simulink model "PTEngineCU"  (Simulink 7.5)
settings: Solver=ode45  StartTime=0.0  StopTime=inf  RelTol=1e-3
PreLoadFcn:
  | Trq_x = [500.0, 600.0, 700.0, 800.0, 1000.0, 2000.0, 3000.0, 4000.0, 4500.0, 5000.0, 6000.0, 7000.0, 8000.0];
  | TrqFull_y = [10.0, 40.0, 70.0, 95.0, 120.0, 145.0, 165.0, 180.0, 185.0, 182.0, 168.0, 130.0, 0.0];
  | 
  | TrqDrag_y = [-10.0, -10.0, -10.0, -10.0, -10.0, -20.0, -30.0, -40.0, -45.0, -50.0, -60.0, -70.0, -80.0];
  | 
  | TrqOpt_y = [0.0, 0.0, 0.0, 0.0, 0.0, 0.0, 0.0, 0.0, 0.0, 0.0, 0.0, 0.0, 0.0];
InitFcn:
  | Trq_x = [500.0, 600.0, 700.0, 800.0, 1000.0, 2000.0, 3000.0, 4000.0, 4500.0, 5000.0, 6000.0, 7000.0, 8000.0];
  | TrqFull_y = [10.0, 40.0, 70.0, 95.0, 120.0, 145.0, 165.0, 180.0, 185.0, 182.0, 168.0, 130.0, 0.0];
  | 
  | TrqDrag_y = [-10.0, -10.0, -10.0, -10.0, -10.0, -20.0, -30.0, -40.0, -45.0, -50.0, -60.0, -70.0, -80.0];
  | 
  | TrqOpt_y = [0.0, 0.0, 0.0, 0.0, 0.0, 0.0, 0.0, 0.0, 0.0, 0.0, 0.0, 0.0, 0.0];
libraries: simulink x8, CarMaker4SL x5
(part 2 of 2)

== system PTEngineCU/CarMaker/IPG Vehicle/CarAndTrailer/Forces/Vehicle Forces ==
  Sync_In : Inport  OutDataType=sfix(16)  OutScaling=2^0
  Bus Creator1 : BusCreator  Inputs=12
  Bus Creator5 : BusCreator  Inputs=13
  Bus Creator8 : BusCreator  Inputs=16
  Demux : Demux  Outputs=16
  Demux1 : Demux  Outputs=12
  Demux5 : Demux  Outputs=13
  Forces : S-Function  FunctionName=CM_Sfun  Parameters='Forces'  EnableBusSupport=off
  Sync_Out : Outport  OutDataType=sfix(16)  OutScaling=2^0
  Car.Virtual : Outport  Port=2  OutDataType=sfix(16)  OutScaling=2^0
  Car.Aero : Outport  Port=3  OutDataType=sfix(16)  OutScaling=2^0
  Car.Load : Outport  Port=4  OutDataType=sfix(16)  OutScaling=2^0
  wires:
  Demux5/7 -> Bus Creator5/7  "car Aero vRes_1 z"
  Demux5/6 -> Bus Creator5/6  "car Aero vRes_1 y"
  Demux5/5 -> Bus Creator5/5  "car Aero vRes_1 x"
  Demux5/4 -> Bus Creator5/4  "Vehicle Wind_vel_0 z"
  Demux5/3 -> Bus Creator5/3  "Vehicle Wind_vel_0 y"
  Demux5/2 -> Bus Creator5/2  "Vehicle Wind_vel_0 x"
  Demux5/1 -> Bus Creator5/1  "Vehicle sRoadAero"
  Demux5/8 -> Bus Creator5/8  "car Aero Frc_1 x"
  Demux5/9 -> Bus Creator5/9  "car Aero Frc_1 y"
  Demux5/10 -> Bus Creator5/10  "car Aero Frc_1 z"
  Demux5/13 -> Bus Creator5/13  "car Aero Trq_1 z"
  Demux5/12 -> Bus Creator5/12  "car Aero Trq_1 y"
  Demux5/11 -> Bus Creator5/11  "car Aero Trq_1 x"
  Forces/4 -> Demux/1
  Demux/12 -> Bus Creator8/12  "Car Load_2 tz"
  Demux/11 -> Bus Creator8/11  "Car Load_2 ty"
  Demux/10 -> Bus Creator8/10  "Car Load_2 tx"
  Demux/9 -> Bus Creator8/9  "Car Load_2 mass"
  Demux/8 -> Bus Creator8/8  "Car Load_1 tz"
  Demux/7 -> Bus Creator8/7  "Car Load_1 ty"
  Demux/6 -> Bus Creator8/6  "Car Load_1 tx"
  Demux/5 -> Bus Creator8/5  "Car Load_1 mass"
  Demux/4 -> Bus Creator8/4  "Car Load_0 tz"
  Demux/3 -> Bus Creator8/3  "Car Load_0 ty"
  Demux/2 -> Bus Creator8/2  "Car Load_0 tx"
  Demux/1 -> Bus Creator8/1  "Car Load_0 mass"
  Bus Creator8/1 -> Car.Load/1
  Bus Creator1/1 -> Car.Virtual/1
  Forces/2 -> Demux1/1
  Forces/3 -> Demux5/1
  Demux1/3 -> Bus Creator1/3  "Car Virtual Frc_1 z"
  Demux1/2 -> Bus Creator1/2  "Car Virtual Frc_1 y"
  Demux1/1 -> Bus Creator1/1  "Car Virtual Frc_1 x"
  Bus Creator5/1 -> Car.Aero/1
  Forces/1 -> Sync_Out/1
  Sync_In/1 -> Forces/1
  Demux1/4 -> Bus Creator1/4  "Car Virtual Frc_0 x"
  Demux1/5 -> Bus Creator1/5  "Car Virtual Frc_0 y"
  Demux1/6 -> Bus Creator1/6  "Car Virtual Frc_0 z"
  Demux1/7 -> Bus Creator1/7  "Car Virtual Trq_1 x"
  Demux1/8 -> Bus Creator1/8  "Car Virtual Trq_1 y"
  Demux1/9 -> Bus Creator1/9  "Car Virtual Trq_1 z"
  Demux1/10 -> Bus Creator1/10  "Car Virtual Trq_0 x"
  Demux1/11 -> Bus Creator1/11  "Car Virtual Trq_0 y"
  Demux1/12 -> Bus Creator1/12  "Car Virtual Trq_0 z"
  Demux/13 -> Bus Creator8/13  "Car Load_3 mass"
  Demux/14 -> Bus Creator8/14  "Car Load_3 tx"
  Demux/15 -> Bus Creator8/15  "Car Load_3 ty"
  Demux/16 -> Bus Creator8/16  "Car Load_3 tz"

== system PTEngineCU/CarMaker/IPG Vehicle/CarAndTrailer/Trailer/CreateBus Car.Hitch.FrcTrq ==
  In1 : Inport  OutDataType=sfix(16)  OutScaling=2^0
  Bus Creator7 : BusCreator  Inputs=6
  Demux7 : Demux  Outputs=6
  Car.Hitch.FrcTrq : Outport  OutDataType=sfix(16)  OutScaling=2^0
  wires:
  Demux7/1 -> Bus Creator7/1  "Car Hitch Frc2Car x"
  Demux7/2 -> Bus Creator7/2  "Car Hitch Frc2Car y"
  Demux7/3 -> Bus Creator7/3  "Car Hitch Frc2Car z"
  Demux7/4 -> Bus Creator7/4  "Car Hitch Trq2Car x"
  Demux7/5 -> Bus Creator7/5  "Car Hitch Trq2Car y"
  Demux7/6 -> Bus Creator7/6  "Car Hitch Trq2Car z"
  Bus Creator7/1 -> Car.Hitch.FrcTrq/1
  In1/1 -> Demux7/1

== system PTEngineCU/CarMaker/IPG Vehicle/CarAndTrailer/Trailer/CreateBus Vhcl.Motion ==
  In1 : Inport  OutDataType=sfix(16)  OutScaling=2^0
  Demux1 : Demux  Outputs=16
  Mux1 : Mux  Inputs=16
  Out1 : Outport  OutDataType=sfix(16)  OutScaling=2^0
  wires:
  Mux1/1 -> Out1/1
  In1/1 -> Demux1/1
  Demux1/16 -> Mux1/16  "Vhcl YawAcc"
  Demux1/15 -> Mux1/15  "Vhcl YawRate"
  Demux1/14 -> Mux1/14  "Vhcl Yaw"
  Demux1/13 -> Mux1/13  "Vhcl PitchAcc"
  Demux1/12 -> Mux1/12  "Vhcl PitchVel"
  Demux1/11 -> Mux1/11  "Vhcl Pitch"
  Demux1/10 -> Mux1/10  "Vhcl RollAcc"
  Demux1/9 -> Mux1/9  "Vhcl RollVel"
  Demux1/8 -> Mux1/8  "Vhcl Roll"
  Demux1/7 -> Mux1/7  "Vhcl Hitch_Pos z"
  Demux1/6 -> Mux1/6  "Vhcl Hitch_Pos y"
  Demux1/5 -> Mux1/5  "Vhcl Hitch_Pos x"
  Demux1/4 -> Mux1/4  "Vhcl sRoadAero"
  Demux1/3 -> Mux1/3  "Vhcl sRoad"
  Demux1/2 -> Mux1/2  "Vhcl Distance"
  Demux1/1 -> Mux1/1  "Vhcl v"

== system PTEngineCU/CarMaker/IPG Vehicle/CarAndTrailer/Trailer/CreateBus Vhcl.PoI ==
  In1 : Inport  OutDataType=sfix(16)  OutScaling=2^0
  Bus Creator3 : BusCreator  Inputs=18
  Demux3 : Demux  Outputs=18
  Out1 : Outport  OutDataType=sfix(16)  OutScaling=2^0
  wires:
  Demux3/1 -> Bus Creator3/1  "Vhcl PoI_Pos x"
  Bus Creator3/1 -> Out1/1
  In1/1 -> Demux3/1
  Demux3/2 -> Bus Creator3/2  "Vhcl PoI_Pos y"
  Demux3/3 -> Bus Creator3/3  "Vhcl PoI_Pos z"
  Demux3/4 -> Bus Creator3/4  "Vhcl PoI_Vel x"
  Demux3/5 -> Bus Creator3/5  "Vhcl PoI_Vel y"
  Demux3/6 -> Bus Creator3/6  "Vhcl PoI_Vel z"
  Demux3/7 -> Bus Creator3/7  "Vhcl PoI_Acc x"
  Demux3/8 -> Bus Creator3/8  "Vhcl PoI_Acc y"
  Demux3/9 -> Bus Creator3/9  "Vhcl PoI_Acc z"
  Demux3/10 -> Bus Creator3/10  "Vhcl PoI_Vel_1 x"
  Demux3/11 -> Bus Creator3/11  "Vhcl PoI_Vel_1 y"
  Demux3/12 -> Bus Creator3/12  "Vhcl PoI_Vel_1 z"
  Demux3/13 -> Bus Creator3/13  "Vhcl PoI_Acc_1 x"
  Demux3/14 -> Bus Creator3/14  "Vhcl PoI_Acc_1 y"
  Demux3/15 -> Bus Creator3/15  "Vhcl PoI_Acc_1 z"
  Demux3/16 -> Bus Creator3/16  "Vhcl PoI_GCS Long"
  Demux3/17 -> Bus Creator3/17  "Vhcl PoI_GCS Lat"
  Demux3/18 -> Bus Creator3/18  "Vhcl PoI_GCS Elev"

== system PTEngineCU/CarMaker/IPG Vehicle/CarAndTrailer/Trailer/CreateBus Vhcl.Steering ==
  In1 : Inport  OutDataType=sfix(16)  OutScaling=2^0
  Bus Creator3 : BusCreator
  Demux : Demux
  Out1 : Outport  OutDataType=sfix(16)  OutScaling=2^0
  wires:
  In1/1 -> Demux/1
  Demux/4 -> Bus Creator3/4  "Vhcl Steering Trq"
  Demux/2 -> Bus Creator3/2  "Vhcl Steering AngVel"
  Demux/3 -> Bus Creator3/3  "Vhcl Steering AngAcc"
  Demux/1 -> Bus Creator3/1  "Vhcl Steering Ang"
  Bus Creator3/1 -> Out1/1

== system PTEngineCU/CarMaker/IPG Vehicle/CarAndTrailer/Trailer/CreateBus Vhcl.Wheel.FL ==
  In1 : Inport  OutDataType=sfix(16)  OutScaling=2^0
  Bus Creator3 : BusCreator  Inputs=14
  Demux3 : Demux  Outputs=14
  Out1 : Outport  OutDataType=sfix(16)  OutScaling=2^0
  wires:
  Demux3/1 -> Bus Creator3/1  "Vhcl Wheel FL t x"
  Bus Creator3/1 -> Out1/1
  In1/1 -> Demux3/1
  Demux3/2 -> Bus Creator3/2  "Vhcl Wheel FL t y"
  Demux3/3 -> Bus Creator3/3  "Vhcl Wheel FL t z"
  Demux3/4 -> Bus Creator3/4  "Vhcl Wheel FL r_zxy x"
  Demux3/5 -> Bus Creator3/5  "Vhcl Wheel FL r_zxy y"
  Demux3/6 -> Bus Creator3/6  "Vhcl Wheel FL r_zxy z"
  Demux3/7 -> Bus Creator3/7  "Vhcl Wheel FL Fx"
  Demux3/8 -> Bus Creator3/8  "Vhcl Wheel FL Fy"
  Demux3/9 -> Bus Creator3/9  "Vhcl Wheel FL Fz"
  Demux3/10 -> Bus Creator3/10  "Vhcl Wheel FL vBelt"
  Demux3/11 -> Bus Creator3/11  "Vhcl Wheel FL LongSlip"
  Demux3/12 -> Bus Creator3/12  "Vhcl Wheel FL SideSlip"
  Demux3/13 -> Bus Creator3/13  "Vhcl Wheel FL Trq_T2W"
  Demux3/14 -> Bus Creator3/14  "Vhcl Wheel FL Trq_WhlBearing"

== system PTEngineCU/CarMaker/IPG Vehicle/CarAndTrailer/Trailer/CreateBus Vhcl.Wheel.FR ==
  In1 : Inport  OutDataType=sfix(16)  OutScaling=2^0
  Bus Creator3 : BusCreator  Inputs=14
  Demux3 : Demux  Outputs=14
  Out1 : Outport  OutDataType=sfix(16)  OutScaling=2^0
  wires:
  Demux3/1 -> Bus Creator3/1  "Vhcl Wheel FR t x"
  Bus Creator3/1 -> Out1/1
  In1/1 -> Demux3/1
  Demux3/2 -> Bus Creator3/2  "Vhcl Wheel FR t y"
  Demux3/3 -> Bus Creator3/3  "Vhcl Wheel FR t z"
  Demux3/4 -> Bus Creator3/4  "Vhcl Wheel FR r_zxy x"
  Demux3/5 -> Bus Creator3/5  "Vhcl Wheel FR r_zxy y"
  Demux3/6 -> Bus Creator3/6  "Vhcl Wheel FR r_zxy z"
  Demux3/7 -> Bus Creator3/7  "Vhcl Wheel FR Fx"
  Demux3/8 -> Bus Creator3/8  "Vhcl Wheel FR Fy"
  Demux3/9 -> Bus Creator3/9  "Vhcl Wheel FR Fz"
  Demux3/10 -> Bus Creator3/10  "Vhcl Wheel FR vBelt"
  Demux3/11 -> Bus Creator3/11  "Vhcl Wheel FR LongSlip"
  Demux3/12 -> Bus Creator3/12  "Vhcl Wheel FR SideSlip"
  Demux3/13 -> Bus Creator3/13  "Vhcl Wheel FR Trq_T2W"
  Demux3/14 -> Bus Creator3/14  "Vhcl Wheel FR Trq_WhlBearing"

== system PTEngineCU/CarMaker/IPG Vehicle/CarAndTrailer/Trailer/CreateBus Vhcl.Wheel.RL ==
  In1 : Inport  OutDataType=sfix(16)  OutScaling=2^0
  Bus Creator3 : BusCreator  Inputs=14
  Demux3 : Demux  Outputs=14
  Out1 : Outport  OutDataType=sfix(16)  OutScaling=2^0
  wires:
  Demux3/1 -> Bus Creator3/1  "Vhcl Wheel RL t x"
  Bus Creator3/1 -> Out1/1
  In1/1 -> Demux3/1
  Demux3/2 -> Bus Creator3/2  "Vhcl Wheel RL t y"
  Demux3/3 -> Bus Creator3/3  "Vhcl Wheel RL t z"
  Demux3/4 -> Bus Creator3/4  "Vhcl Wheel RL r_zxy x"
  Demux3/5 -> Bus Creator3/5  "Vhcl Wheel RL r_zxy y"
  Demux3/6 -> Bus Creator3/6  "Vhcl Wheel RL r_zxy z"
  Demux3/7 -> Bus Creator3/7  "Vhcl Wheel RL Fx"
  Demux3/8 -> Bus Creator3/8  "Vhcl Wheel RL Fy"
  Demux3/9 -> Bus Creator3/9  "Vhcl Wheel RL Fz"
  Demux3/10 -> Bus Creator3/10  "Vhcl Wheel RL vBelt"
  Demux3/11 -> Bus Creator3/11  "Vhcl Wheel RL LongSlip"
  Demux3/12 -> Bus Creator3/12  "Vhcl Wheel RL SideSlip"
  Demux3/13 -> Bus Creator3/13  "Vhcl Wheel RL Trq_T2W"
  Demux3/14 -> Bus Creator3/14  "Vhcl Wheel RL Trq_WhlBearing"

== system PTEngineCU/CarMaker/IPG Vehicle/CarAndTrailer/Trailer/CreateBus Vhcl.Wheel.RR ==
  In1 : Inport  OutDataType=sfix(16)  OutScaling=2^0
  Bus Creator3 : BusCreator  Inputs=14
  Demux3 : Demux  Outputs=14
  Out1 : Outport  OutDataType=sfix(16)  OutScaling=2^0
  wires:
  Demux3/1 -> Bus Creator3/1  "Vhcl Wheel RR t x"
  Bus Creator3/1 -> Out1/1
  In1/1 -> Demux3/1
  Demux3/2 -> Bus Creator3/2  "Vhcl Wheel RR t y"
  Demux3/3 -> Bus Creator3/3  "Vhcl Wheel RR t z"
  Demux3/4 -> Bus Creator3/4  "Vhcl Wheel RR r_zxy x"
  Demux3/5 -> Bus Creator3/5  "Vhcl Wheel RR r_zxy y"
  Demux3/6 -> Bus Creator3/6  "Vhcl Wheel RR r_zxy z"
  Demux3/7 -> Bus Creator3/7  "Vhcl Wheel RR Fx"
  Demux3/8 -> Bus Creator3/8  "Vhcl Wheel RR Fy"
  Demux3/9 -> Bus Creator3/9  "Vhcl Wheel RR Fz"
  Demux3/10 -> Bus Creator3/10  "Vhcl Wheel RR vBelt"
  Demux3/11 -> Bus Creator3/11  "Vhcl Wheel RR LongSlip"
  Demux3/12 -> Bus Creator3/12  "Vhcl Wheel RR SideSlip"
  Demux3/13 -> Bus Creator3/13  "Vhcl Wheel RR Trq_T2W"
  Demux3/14 -> Bus Creator3/14  "Vhcl Wheel RR Trq_WhlBearing"

== system PTEngineCU/CarMaker/IPG Vehicle/PowerTrain/ECU Example/CreateBus ECU_IF Output ==
  In : Inport
  BusCreator : BusCreator  Inputs=7
  Demux : Demux  Outputs=7
  Out : Outport
  wires:
  In/1 -> Demux/1
  BusCreator/1 -> Out/1
  Demux/1 -> BusCreator/1  "ECU_Out Status"
  Demux/2 -> BusCreator/2  "ECU_Out FuelCutOff"
  Demux/3 -> BusCreator/3  "ECU_Out Engine_on"
  Demux/4 -> BusCreator/4  "ECU_Out Load"
  Demux/5 -> BusCreator/5  "ECU_Out TrqDrag"
  Demux/6 -> BusCreator/6  "ECU_Out TrqFull"
  Demux/7 -> BusCreator/7  "ECU_Out TrqOpt"

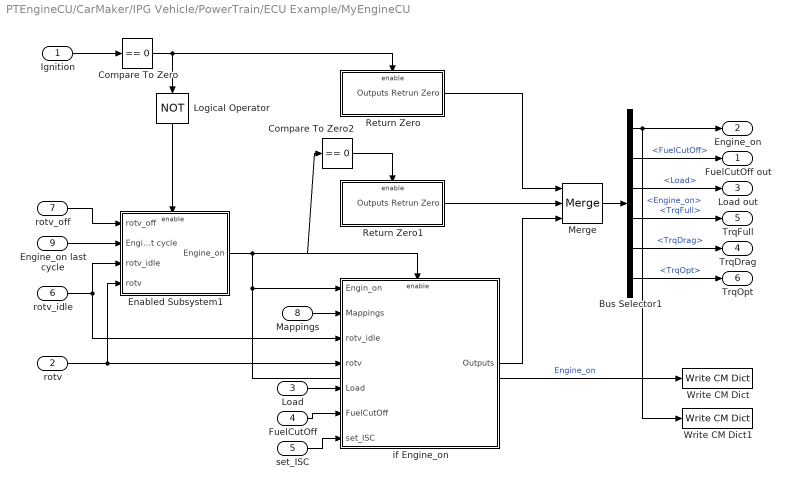
== system PTEngineCU/CarMaker/IPG Vehicle/PowerTrain/ECU Example/MyEngineCU ==
  Ignition : Inport  OutDataType=sfix(16)  OutScaling=2^0
  rotv : Inport  Port=2  OutDataType=sfix(16)  OutScaling=2^0
  Load : Inport  Port=3  OutDataType=sfix(16)  OutScaling=2^0
  FuelCutOff : Inport  Port=4  OutDataType=sfix(16)  OutScaling=2^0
  set_ISC : Inport  Port=5  OutDataType=sfix(16)  OutScaling=2^0
  rotv_idle : Inport  Port=6  OutDataType=sfix(16)  OutScaling=2^0
  rotv_off : Inport  Port=7  OutDataType=sfix(16)  OutScaling=2^0
  Mappings : Inport  Port=8  OutDataType=sfix(16)  OutScaling=2^0
  Engine_on last cycle : Inport  Port=9  OutDataType=sfix(16)  OutScaling=2^0
  Bus Selector1 : BusSelector  OutputSignals=Engine_on,FuelCutOff,Load,TrqFull,TrqDrag,TrqOpt
  Compare To Zero : simulink/Logic and Bit Operations/Compare To Zero  SystemSampleTime=-1  relop===  LogicOutDataTypeMode=uint8  ZeroCross=off
  Compare To Zero2 : simulink/Logic and Bit Operations/Compare To Zero  SystemSampleTime=-1  relop===  LogicOutDataTypeMode=uint8  ZeroCross=off
  Enabled Subsystem1 : Subsystem  TreatAsAtomicUnit=on
  Logical Operator : Logic  Operator=NOT  AllPortsSameDT=off  OutDataTypeMode=boolean  OutDataTypeStr=boolean
  Merge : Merge  Inputs=3
  Return Zero : Subsystem  TreatAsAtomicUnit=on
  Return Zero1 : Subsystem  TreatAsAtomicUnit=on
  Write CM Dict : CarMaker4SL/Write CM Dict  xname=UserOut_00  xsync=off
  Write CM Dict1 : CarMaker4SL/Write CM Dict  xname=UserOut_01  xsync=off
  if Engine_on : Subsystem  TreatAsAtomicUnit=on
  FuelCutOff out : Outport  OutDataType=sfix(16)  OutScaling=2^0
  Engine_on : Outport  Port=2  OutDataType=sfix(16)  OutScaling=2^0
  Load out : Outport  Port=3  OutDataType=sfix(16)  OutScaling=2^0
  TrqDrag : Outport  Port=4  OutDataType=sfix(16)  OutScaling=2^0
  TrqFull : Outport  Port=5  OutDataType=sfix(16)  OutScaling=2^0
  TrqOpt : Outport  Port=6  OutDataType=sfix(16)  OutScaling=2^0
  wires:
  Ignition/1 -> Compare To Zero/1
  Compare To Zero/1 -> Logical Operator/1, Return Zero/Enable
  Logical Operator/1 -> Enabled Subsystem1/Enable
  Enabled Subsystem1/1(Engine_on) -> Compare To Zero2/1, if Engine_on/Enable, if Engine_on/1(Engin_on), Write CM Dict/1  "Engine_on"
  Mappings/1 -> if Engine_on/2(Mappings)
  rotv/1 -> Enabled Subsystem1/4(rotv), if Engine_on/4(rotv)
  rotv_idle/1 -> Enabled Subsystem1/3(rotv_idle), if Engine_on/3(rotv_idle)
  rotv_off/1 -> Enabled Subsystem1/1(rotv_off)
  Engine_on last cycle/1 -> Enabled Subsystem1/2(Engine_on last cycle)
  Load/1 -> if Engine_on/5(Load)
  FuelCutOff/1 -> if Engine_on/6(FuelCutOff)
  set_ISC/1 -> if Engine_on/7(set_ISC)
  Return Zero/1(Outputs Retrun Zero) -> Merge/1
  Merge/1 -> Bus Selector1/1
  Bus Selector1/1 -> Engine_on/1, Write CM Dict1/1  "<Engine_on>"
  Bus Selector1/3 -> Load out/1  "<Load>"
  Bus Selector1/5 -> TrqDrag/1  "<TrqDrag>"
  Bus Selector1/4 -> TrqFull/1  "<TrqFull>"
  Bus Selector1/6 -> TrqOpt/1  "<TrqOpt>"
  Bus Selector1/2 -> FuelCutOff out/1  "<FuelCutOff>"
  Compare To Zero2/1 -> Return Zero1/Enable
  Return Zero1/1(Outputs Retrun Zero) -> Merge/2
  if Engine_on/1(Outputs) -> Merge/3

== system PTEngineCU/CarMaker/IPG Vehicle/PowerTrain/ECU Example/PTEngineCU_In ==
  Sync_In : Inport
  CreateBus ECU_CfgIF : Subsystem
  CreateBus ECU_IF Input : Subsystem
  CreateBus PTEngineCU_In : BusCreator  Inputs=2
  S-Function : S-Function  FunctionName=cm_ptenginecu_in  EnableBusSupport=off
  PTEngineCU_In : Outport
  wires:
  Sync_In/1 -> S-Function/1
  CreateBus PTEngineCU_In/1 -> PTEngineCU_In/1
  S-Function/1 -> CreateBus ECU_CfgIF/1(In)
  CreateBus ECU_CfgIF/1(Out) -> CreateBus PTEngineCU_In/1  "ECU_CfgIF"
  S-Function/2 -> CreateBus ECU_IF Input/1(In)
  CreateBus ECU_IF Input/1(Out) -> CreateBus PTEngineCU_In/2  "ECU_IF Input"

== system PTEngineCU/CarMaker/IPG Vehicle/PowerTrain/ECU Example/PTEngineCU_Out ==
  ECU_IF Output : Inport
  S-Function : S-Function  FunctionName=cm_ptenginecu_out  EnableBusSupport=off
  wires:
  ECU_IF Output/1 -> S-Function/1

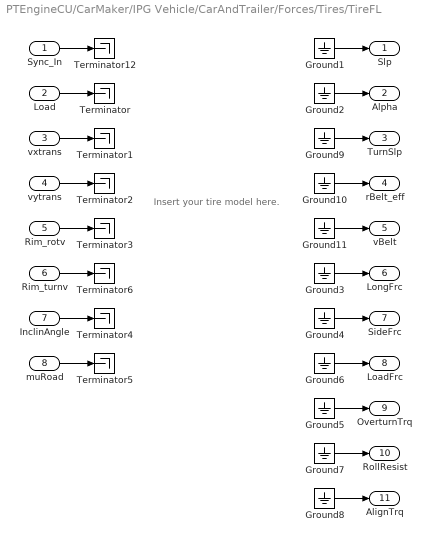
== system PTEngineCU/CarMaker/IPG Vehicle/CarAndTrailer/Forces/Tires/TireFL ==
  note: Insert your tire model here.
  Sync_In : Inport  OutDataType=sfix(16)  OutScaling=2^0
  Load : Inport  Port=2  OutDataType=sfix(16)  OutScaling=2^0
  vxtrans : Inport  Port=3  OutDataType=sfix(16)  OutScaling=2^0
  vytrans : Inport  Port=4  OutDataType=sfix(16)  OutScaling=2^0
  Rim_rotv : Inport  Port=5  OutDataType=sfix(16)  OutScaling=2^0
  Rim_turnv : Inport  Port=6  OutDataType=sfix(16)  OutScaling=2^0
  InclinAngle : Inport  Port=7  OutDataType=sfix(16)  OutScaling=2^0
  muRoad : Inport  Port=8  OutDataType=sfix(16)  OutScaling=2^0
  Ground{1..11} (11 alike) : Ground
  Terminator{,1..6,12} (8 alike) : Terminator
  Slp : Outport  OutDataType=sfix(16)  OutScaling=2^0
  Alpha : Outport  Port=2  OutDataType=sfix(16)  OutScaling=2^0
  TurnSlp : Outport  Port=3  OutDataType=sfix(16)  OutScaling=2^0
  rBelt_eff : Outport  Port=4  OutDataType=sfix(16)  OutScaling=2^0
  vBelt : Outport  Port=5  OutDataType=sfix(16)  OutScaling=2^0
  LongFrc : Outport  Port=6  OutDataType=sfix(16)  OutScaling=2^0
  SideFrc : Outport  Port=7  OutDataType=sfix(16)  OutScaling=2^0
  LoadFrc : Outport  Port=8  OutDataType=sfix(16)  OutScaling=2^0
  OverturnTrq : Outport  Port=9  OutDataType=sfix(16)  OutScaling=2^0
  RollResist : Outport  Port=10  OutDataType=sfix(16)  OutScaling=2^0
  AlignTrq : Outport  Port=11  OutDataType=sfix(16)  OutScaling=2^0
  wires:
  Ground11/1 -> vBelt/1
  Ground10/1 -> rBelt_eff/1
  Ground9/1 -> TurnSlp/1
  Rim_turnv/1 -> Terminator6/1
  Sync_In/1 -> Terminator12/1
  Ground2/1 -> Alpha/1
  Ground3/1 -> LongFrc/1
  Ground4/1 -> SideFrc/1
  Ground5/1 -> OverturnTrq/1
  vxtrans/1 -> Terminator1/1
  vytrans/1 -> Terminator2/1
  Rim_rotv/1 -> Terminator3/1
  InclinAngle/1 -> Terminator4/1
  muRoad/1 -> Terminator5/1
  Load/1 -> Terminator/1
  Ground1/1 -> Slp/1
  Ground6/1 -> LoadFrc/1
  Ground7/1 -> RollResist/1
  Ground8/1 -> AlignTrq/1

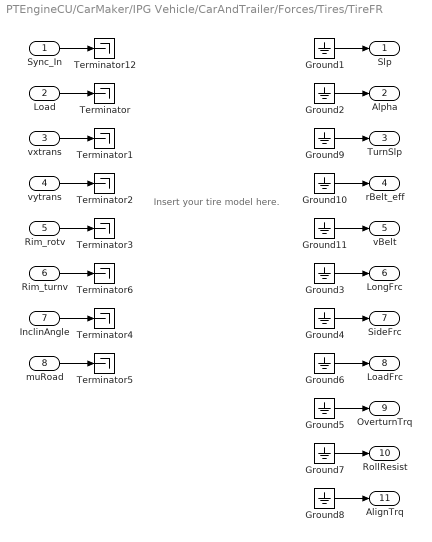
== system PTEngineCU/CarMaker/IPG Vehicle/CarAndTrailer/Forces/Tires/TireFR ==
  note: Insert your tire model here.
  Sync_In : Inport  OutDataType=sfix(16)  OutScaling=2^0
  Load : Inport  Port=2  OutDataType=sfix(16)  OutScaling=2^0
  vxtrans : Inport  Port=3  OutDataType=sfix(16)  OutScaling=2^0
  vytrans : Inport  Port=4  OutDataType=sfix(16)  OutScaling=2^0
  Rim_rotv : Inport  Port=5  OutDataType=sfix(16)  OutScaling=2^0
  Rim_turnv : Inport  Port=6  OutDataType=sfix(16)  OutScaling=2^0
  InclinAngle : Inport  Port=7  OutDataType=sfix(16)  OutScaling=2^0
  muRoad : Inport  Port=8  OutDataType=sfix(16)  OutScaling=2^0
  Ground{1..11} (11 alike) : Ground
  Terminator{,1..6,12} (8 alike) : Terminator
  Slp : Outport  OutDataType=sfix(16)  OutScaling=2^0
  Alpha : Outport  Port=2  OutDataType=sfix(16)  OutScaling=2^0
  TurnSlp : Outport  Port=3  OutDataType=sfix(16)  OutScaling=2^0
  rBelt_eff : Outport  Port=4  OutDataType=sfix(16)  OutScaling=2^0
  vBelt : Outport  Port=5  OutDataType=sfix(16)  OutScaling=2^0
  LongFrc : Outport  Port=6  OutDataType=sfix(16)  OutScaling=2^0
  SideFrc : Outport  Port=7  OutDataType=sfix(16)  OutScaling=2^0
  LoadFrc : Outport  Port=8  OutDataType=sfix(16)  OutScaling=2^0
  OverturnTrq : Outport  Port=9  OutDataType=sfix(16)  OutScaling=2^0
  RollResist : Outport  Port=10  OutDataType=sfix(16)  OutScaling=2^0
  AlignTrq : Outport  Port=11  OutDataType=sfix(16)  OutScaling=2^0
  wires:
  Ground11/1 -> vBelt/1
  Ground10/1 -> rBelt_eff/1
  Ground9/1 -> TurnSlp/1
  Rim_turnv/1 -> Terminator6/1
  Sync_In/1 -> Terminator12/1
  Ground2/1 -> Alpha/1
  Ground3/1 -> LongFrc/1
  Ground4/1 -> SideFrc/1
  Ground5/1 -> OverturnTrq/1
  vxtrans/1 -> Terminator1/1
  vytrans/1 -> Terminator2/1
  Rim_rotv/1 -> Terminator3/1
  InclinAngle/1 -> Terminator4/1
  muRoad/1 -> Terminator5/1
  Load/1 -> Terminator/1
  Ground1/1 -> Slp/1
  Ground6/1 -> LoadFrc/1
  Ground7/1 -> RollResist/1
  Ground8/1 -> AlignTrq/1

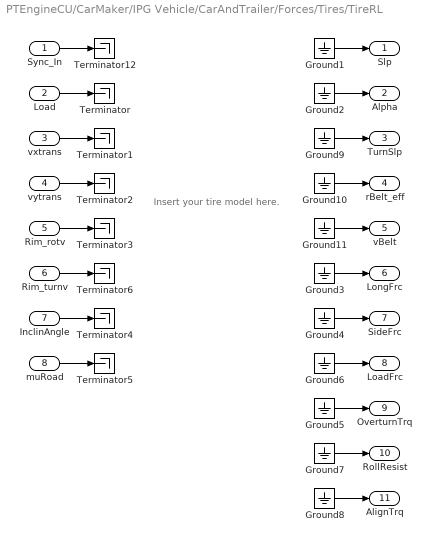
== system PTEngineCU/CarMaker/IPG Vehicle/CarAndTrailer/Forces/Tires/TireRL ==
  note: Insert your tire model here.
  Sync_In : Inport  OutDataType=sfix(16)  OutScaling=2^0
  Load : Inport  Port=2  OutDataType=sfix(16)  OutScaling=2^0
  vxtrans : Inport  Port=3  OutDataType=sfix(16)  OutScaling=2^0
  vytrans : Inport  Port=4  OutDataType=sfix(16)  OutScaling=2^0
  Rim_rotv : Inport  Port=5  OutDataType=sfix(16)  OutScaling=2^0
  Rim_turnv : Inport  Port=6  OutDataType=sfix(16)  OutScaling=2^0
  InclinAngle : Inport  Port=7  OutDataType=sfix(16)  OutScaling=2^0
  muRoad : Inport  Port=8  OutDataType=sfix(16)  OutScaling=2^0
  Ground{1..11} (11 alike) : Ground
  Terminator{,1..6,12} (8 alike) : Terminator
  Slp : Outport  OutDataType=sfix(16)  OutScaling=2^0
  Alpha : Outport  Port=2  OutDataType=sfix(16)  OutScaling=2^0
  TurnSlp : Outport  Port=3  OutDataType=sfix(16)  OutScaling=2^0
  rBelt_eff : Outport  Port=4  OutDataType=sfix(16)  OutScaling=2^0
  vBelt : Outport  Port=5  OutDataType=sfix(16)  OutScaling=2^0
  LongFrc : Outport  Port=6  OutDataType=sfix(16)  OutScaling=2^0
  SideFrc : Outport  Port=7  OutDataType=sfix(16)  OutScaling=2^0
  LoadFrc : Outport  Port=8  OutDataType=sfix(16)  OutScaling=2^0
  OverturnTrq : Outport  Port=9  OutDataType=sfix(16)  OutScaling=2^0
  RollResist : Outport  Port=10  OutDataType=sfix(16)  OutScaling=2^0
  AlignTrq : Outport  Port=11  OutDataType=sfix(16)  OutScaling=2^0
  wires:
  Ground11/1 -> vBelt/1
  Ground10/1 -> rBelt_eff/1
  Ground9/1 -> TurnSlp/1
  Rim_turnv/1 -> Terminator6/1
  Sync_In/1 -> Terminator12/1
  Ground2/1 -> Alpha/1
  Ground3/1 -> LongFrc/1
  Ground4/1 -> SideFrc/1
  Ground5/1 -> OverturnTrq/1
  vxtrans/1 -> Terminator1/1
  vytrans/1 -> Terminator2/1
  Rim_rotv/1 -> Terminator3/1
  InclinAngle/1 -> Terminator4/1
  muRoad/1 -> Terminator5/1
  Load/1 -> Terminator/1
  Ground1/1 -> Slp/1
  Ground6/1 -> LoadFrc/1
  Ground7/1 -> RollResist/1
  Ground8/1 -> AlignTrq/1

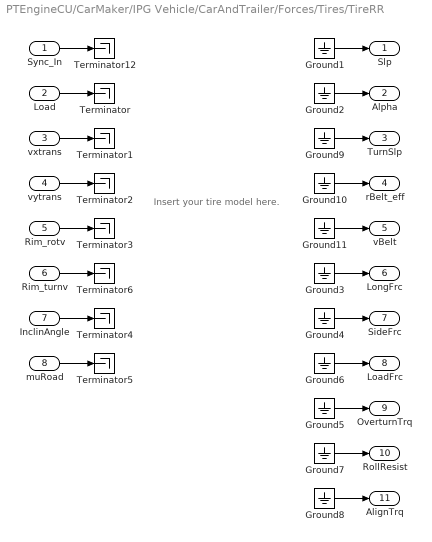
== system PTEngineCU/CarMaker/IPG Vehicle/CarAndTrailer/Forces/Tires/TireRR ==
  note: Insert your tire model here.
  Sync_In : Inport  OutDataType=sfix(16)  OutScaling=2^0
  Load : Inport  Port=2  OutDataType=sfix(16)  OutScaling=2^0
  vxtrans : Inport  Port=3  OutDataType=sfix(16)  OutScaling=2^0
  vytrans : Inport  Port=4  OutDataType=sfix(16)  OutScaling=2^0
  Rim_rotv : Inport  Port=5  OutDataType=sfix(16)  OutScaling=2^0
  Rim_turnv : Inport  Port=6  OutDataType=sfix(16)  OutScaling=2^0
  InclinAngle : Inport  Port=7  OutDataType=sfix(16)  OutScaling=2^0
  muRoad : Inport  Port=8  OutDataType=sfix(16)  OutScaling=2^0
  Ground{1..11} (11 alike) : Ground
  Terminator{,1..6,12} (8 alike) : Terminator
  Slp : Outport  OutDataType=sfix(16)  OutScaling=2^0
  Alpha : Outport  Port=2  OutDataType=sfix(16)  OutScaling=2^0
  TurnSlp : Outport  Port=3  OutDataType=sfix(16)  OutScaling=2^0
  rBelt_eff : Outport  Port=4  OutDataType=sfix(16)  OutScaling=2^0
  vBelt : Outport  Port=5  OutDataType=sfix(16)  OutScaling=2^0
  LongFrc : Outport  Port=6  OutDataType=sfix(16)  OutScaling=2^0
  SideFrc : Outport  Port=7  OutDataType=sfix(16)  OutScaling=2^0
  LoadFrc : Outport  Port=8  OutDataType=sfix(16)  OutScaling=2^0
  OverturnTrq : Outport  Port=9  OutDataType=sfix(16)  OutScaling=2^0
  RollResist : Outport  Port=10  OutDataType=sfix(16)  OutScaling=2^0
  AlignTrq : Outport  Port=11  OutDataType=sfix(16)  OutScaling=2^0
  wires:
  Ground11/1 -> vBelt/1
  Ground10/1 -> rBelt_eff/1
  Ground9/1 -> TurnSlp/1
  Rim_turnv/1 -> Terminator6/1
  Sync_In/1 -> Terminator12/1
  Ground2/1 -> Alpha/1
  Ground3/1 -> LongFrc/1
  Ground4/1 -> SideFrc/1
  Ground5/1 -> OverturnTrq/1
  vxtrans/1 -> Terminator1/1
  vytrans/1 -> Terminator2/1
  Rim_rotv/1 -> Terminator3/1
  InclinAngle/1 -> Terminator4/1
  muRoad/1 -> Terminator5/1
  Load/1 -> Terminator/1
  Ground1/1 -> Slp/1
  Ground6/1 -> LoadFrc/1
  Ground7/1 -> RollResist/1
  Ground8/1 -> AlignTrq/1

== system PTEngineCU/CarMaker/IPG Vehicle/PowerTrain/ECU Example/MyEngineCU/Enabled Subsystem1 ==
  rotv_off : Inport  OutDataType=sfix(16)  OutScaling=2^0
  Engine_on last cycle : Inport  Port=2  OutDataType=sfix(16)  OutScaling=2^0
  rotv_idle : Inport  Port=3  OutDataType=sfix(16)  OutScaling=2^0
  rotv : Inport  Port=4  OutDataType=sfix(16)  OutScaling=2^0
  Enable : EnablePort
  Engine off : Subsystem  TreatAsAtomicUnit=on
  Engine on : Subsystem  TreatAsAtomicUnit=on
  Engine on? : If  NumInputs=3  IfExpression=u1 > u2  ElseIfExpressions=u1 < u3
  If Action Subsystem2 : Subsystem  TreatAsAtomicUnit=on
  Merge : Merge  Inputs=3
  Engine_on : Outport  OutDataType=sfix(16)  OutScaling=2^0
  wires:
  rotv/1 -> Engine on?/1
  rotv_idle/1 -> Engine on?/2
  rotv_off/1 -> Engine on?/3
  Engine on?/1 -> Engine on/Action
  Engine on?/2 -> Engine off/Action
  Engine on?/3 -> If Action Subsystem2/Action
  Engine_on last cycle/1 -> If Action Subsystem2/1(Engine_on last cycle)
  Merge/1 -> Engine_on/1
  If Action Subsystem2/1(Engine_on) -> Merge/3
  Engine on/1(Engine_on) -> Merge/1
  Engine off/1(Engine_off) -> Merge/2

== system PTEngineCU/CarMaker/IPG Vehicle/PowerTrain/ECU Example/MyEngineCU/Return Zero ==
  Enable : EnablePort
  Bus Creator : BusCreator  Inputs=6
  Constant : Constant  Value=0  OutDataType=sfix(16)  OutScaling=2^0
  Constant1 : Constant  Value=0  OutDataType=sfix(16)  OutScaling=2^0
  Constant{2..5} (4 alike) : Constant  Value=0.0  OutDataType=sfix(16)  OutScaling=2^0
  Outputs Retrun Zero : Outport  SampleTime=0.001  OutDataType=sfix(16)  OutScaling=2^0  InitialOutput=0
  wires:
  Bus Creator/1 -> Outputs Retrun Zero/1
  Constant/1 -> Bus Creator/1  "Engine_on"
  Constant1/1 -> Bus Creator/2  "FuelCutOff"
  Constant2/1 -> Bus Creator/3  "Load"
  Constant3/1 -> Bus Creator/4  "TrqFull"
  Constant4/1 -> Bus Creator/5  "TrqDrag"
  Constant5/1 -> Bus Creator/6  "TrqOpt"

== system PTEngineCU/CarMaker/IPG Vehicle/PowerTrain/ECU Example/MyEngineCU/Return Zero1 ==
  Enable : EnablePort
  Bus Creator : BusCreator  Inputs=6
  Constant : Constant  Value=0  OutDataType=sfix(16)  OutScaling=2^0
  Constant1 : Constant  Value=0  OutDataType=sfix(16)  OutScaling=2^0
  Constant{2..5} (4 alike) : Constant  Value=0.0  OutDataType=sfix(16)  OutScaling=2^0
  Outputs Retrun Zero : Outport  SampleTime=0.001  OutDataType=sfix(16)  OutScaling=2^0  InitialOutput=0
  wires:
  Constant5/1 -> Bus Creator/6  "TrqOpt"
  Constant4/1 -> Bus Creator/5  "TrqDrag"
  Constant3/1 -> Bus Creator/4  "TrqFull"
  Constant2/1 -> Bus Creator/3  "Load"
  Constant1/1 -> Bus Creator/2  "FuelCutOff"
  Constant/1 -> Bus Creator/1  "Engine_on"
  Bus Creator/1 -> Outputs Retrun Zero/1

== system PTEngineCU/CarMaker/IPG Vehicle/PowerTrain/ECU Example/MyEngineCU/if Engine_on ==
  Engin_on : Inport  OutDataType=sfix(16)  OutScaling=2^0
  Mappings : Inport  Port=2  OutDataType=sfix(16)  OutScaling=2^0
  rotv_idle : Inport  Port=3  OutDataType=sfix(16)  OutScaling=2^0
  rotv : Inport  Port=4  OutDataType=sfix(16)  OutScaling=2^0
  Load : Inport  Port=5  OutDataType=sfix(16)  OutScaling=2^0
  FuelCutOff : Inport  Port=6  OutDataType=sfix(16)  OutScaling=2^0
  set_ISC : Inport  Port=7  OutDataType=sfix(16)  OutScaling=2^0
  Enable : EnablePort
  == NOTSET : simulink/Logic and Bit Operations/Compare To Constant  SystemSampleTime=-1  relop===  const=-9999  LogicOutDataTypeMode=uint8  ZeroCross=off
  Bus Creator : BusCreator  Inputs=6
  Bus Selector4 : BusSelector  OutputSignals=TrqFull,TrqDrag,TrqOpt
  Constant : Constant  Value=0.0  OutDataType=sfix(16)  OutScaling=2^0
  FuelCutOff Function : Subsystem
  Gain : Gain  ParameterDataType=sfix(16)  ParameterScaling=2^0  OutDataType=sfix(16)  OutScaling=2^0
  Idle Speed Control : Subsystem
  Switch : Switch  Criteria=u2 ~= 0  OutDataType=sfix(16)  OutScaling=2^0
  TrqFull & TrqDrag & TrqOpt : Subsystem
  Outputs : Outport  OutDataType=sfix(16)  OutScaling=2^0
  wires:
  Bus Creator/1 -> Outputs/1
  Mappings/1 -> TrqFull & TrqDrag & TrqOpt/2(Mappings)
  rotv/1 -> TrqFull & TrqDrag & TrqOpt/1(rotv), FuelCutOff Function/3(rotv), Idle Speed Control/4(rotv)
  Load/1 -> == NOTSET/1, Switch/3
  == NOTSET/1 -> Switch/2
  Constant/1 -> Switch/1
  TrqFull & TrqDrag & TrqOpt/1(Trg) -> Bus Selector4/1
  FuelCutOff/1 -> FuelCutOff Function/1(FuelCutOff)
  Idle Speed Control/1(Load_out) -> FuelCutOff Function/2(Load)
  rotv_idle/1 -> Idle Speed Control/1(rotv_idle)
  set_ISC/1 -> Idle Speed Control/2(set_ISC)
  Switch/1 -> Idle Speed Control/3(Load)  "Load"
  Engin_on/1 -> Gain/1
  FuelCutOff Function/1(FuelCutOff1) -> Bus Creator/2  "FuelCutOff"
  FuelCutOff Function/2(Load1) -> Bus Creator/3  "Load"
  Bus Selector4/1 -> Bus Creator/4  "<TrqFull>"
  Bus Selector4/2 -> Bus Creator/5  "<TrqDrag>"
  Bus Selector4/3 -> Bus Creator/6  "<TrqOpt>"
  Gain/1 -> Bus Creator/1  "Engine_on"

== system PTEngineCU/CarMaker/IPG Vehicle/PowerTrain/ECU Example/PTEngineCU_In/CreateBus ECU_CfgIF ==
  In : Inport
  BusCreator : BusCreator
  Demux : Demux
  Out : Outport
  wires:
  In/1 -> Demux/1
  BusCreator/1 -> Out/1
  Demux/1 -> BusCreator/1  "ECU_Cfg rotv_off"
  Demux/2 -> BusCreator/2  "ECU_Cfg rotv_max"
  Demux/3 -> BusCreator/3  "ECU_Cfg rotv_idle"
  Demux/4 -> BusCreator/4  "ECU_Cfg rotv_opt"

== system PTEngineCU/CarMaker/IPG Vehicle/PowerTrain/ECU Example/PTEngineCU_In/CreateBus ECU_IF Input ==
  In : Inport
  BusCreator : BusCreator  Inputs=10
  Demux : Demux  Outputs=10
  Out : Outport
  wires:
  In/1 -> Demux/1
  BusCreator/1 -> Out/1
  Demux/1 -> BusCreator/1  "ECU Ignition"
  Demux/2 -> BusCreator/2  "ECU set_ISC"
  Demux/3 -> BusCreator/3  "ECU FuelCutOff"
  Demux/4 -> BusCreator/4  "ECU Load"
  Demux/5 -> BusCreator/5  "ECU Trq_trg"
  Demux/6 -> BusCreator/6  "ECU Trq"
  Demux/7 -> BusCreator/7  "ECU rotv_trg"
  Demux/8 -> BusCreator/8  "ECU rotv"
  Demux/9 -> BusCreator/9  "ECU rot"
  Demux/10 -> BusCreator/10  "ECU FuelFlow"

== system PTEngineCU/CarMaker/IPG Vehicle/PowerTrain/ECU Example/MyEngineCU/Enabled Subsystem1/Engine off ==
  Action Port : ActionPort  ActionType=elseif
  Constant : Constant  Value=0  OutDataType=sfix(16)  OutScaling=2^0
  Engine_off : Outport  OutDataType=sfix(16)  OutScaling=2^0  InitialOutput=0
  wires:
  Constant/1 -> Engine_off/1

== system PTEngineCU/CarMaker/IPG Vehicle/PowerTrain/ECU Example/MyEngineCU/Enabled Subsystem1/Engine on ==
  Action Port : ActionPort  ActionType=then
  Constant : Constant  OutDataType=sfix(16)  OutScaling=2^0
  Engine_on : Outport  OutDataType=sfix(16)  OutScaling=2^0  InitialOutput=1
  wires:
  Constant/1 -> Engine_on/1

== system PTEngineCU/CarMaker/IPG Vehicle/PowerTrain/ECU Example/MyEngineCU/Enabled Subsystem1/If Action Subsystem2 ==
  Engine_on last cycle : Inport  OutDataType=sfix(16)  OutScaling=2^0
  Action Port : ActionPort  ActionType=else
  Engine_on : Outport  OutDataType=sfix(16)  OutScaling=2^0
  wires:
  Engine_on last cycle/1 -> Engine_on/1

== system PTEngineCU/CarMaker/IPG Vehicle/PowerTrain/ECU Example/MyEngineCU/if Engine_on/FuelCutOff Function ==
  FuelCutOff : Inport  OutDataType=sfix(16)  OutScaling=2^0
  Load : Inport  Port=2
  rotv : Inport  Port=3
  If : If  IfExpression=u1 == 1  ElseIfExpressions=u1 == -99999
  If Action Subsystem : Subsystem  TreatAsAtomicUnit=on
  If Action Subsystem1 : Subsystem  TreatAsAtomicUnit=on
  If Action Subsystem2 : Subsystem  TreatAsAtomicUnit=on
  Merge : Merge  Inputs=3
  Merge1 : Merge  Inputs=3
  Read CM Parameter : CarMaker4SL/Read CM Parameter  xfile=Vehicle  xkey=PowerTrain.ECU.FuelCutOff  xnout=1  xdefaults=1600  xmuxed=on
  rpm2radsec : Gain  Gain=0.104719755  ParameterDataType=sfix(16)  ParameterScaling=2^0  OutDataType=sfix(16)  OutScaling=2^0
  FuelCutOff1 : Outport
  Load1 : Outport  Port=2
  wires:
  If/3 -> If Action Subsystem1/Action
  If/2 -> If Action Subsystem2/Action
  If/1 -> If Action Subsystem/Action
  If Action Subsystem/1(FuelCutOff out) -> Merge/1
  If Action Subsystem1/1(FuelCutOff out) -> Merge/2
  If Action Subsystem2/1(FuelCutOff out) -> Merge/3
  If Action Subsystem2/2(Load out) -> Merge1/3
  If Action Subsystem1/2(Load out) -> Merge1/2
  If Action Subsystem/2(Load out) -> Merge1/1
  rotv/1 -> If Action Subsystem2/2(rotv)
  Read CM Parameter/1 -> rpm2radsec/1
  Merge/1 -> FuelCutOff1/1
  Merge1/1 -> Load1/1
  FuelCutOff/1 -> If/1, If Action Subsystem/1(FuelCutOff), If Action Subsystem1/1(FuelCutOff)
  Load/1 -> If Action Subsystem1/2(Load), If Action Subsystem2/1(Load)  "Load"
  rpm2radsec/1 -> If Action Subsystem2/3(nFuelCutOff)

== system PTEngineCU/CarMaker/IPG Vehicle/PowerTrain/ECU Example/MyEngineCU/if Engine_on/Idle Speed Control ==
  rotv_idle : Inport  OutDataType=sfix(16)  OutScaling=2^0
  set_ISC : Inport  Port=2  OutDataType=sfix(16)  OutScaling=2^0
  Load : Inport  Port=3
  rotv : Inport  Port=4
  Bus Creator1 : BusCreator  Inputs=2
  Bus Creator2 : BusCreator  Inputs=2
  Bus Selector : BusSelector  OutputSignals=Load_I,Load
  Constant2 : Constant  Value=0.0  OutDataType=sfix(16)  OutScaling=2^0
  Load Copy : InportShadow  Port=3
  Load Copy2 : InportShadow  Port=3
  Memory1 : Memory  InheritSampleTime=on
  PI : Subsystem
  Saturation : Saturate  UpperLimit=1  LowerLimit=0  OutDataType=sfix(16)  OutScaling=2^0
  Subtract : Sum  Inputs=+-  OutDataType=sfix(16)  OutScaling=2^-10
  Switch1 : Switch  Criteria=u2 ~= 0  OutDataType=sfix(16)  OutScaling=2^0
  Switch2 : Switch  Criteria=u2 ~= 0  OutDataType=sfix(16)  OutScaling=2^0
  if condition : Subsystem
  Load_out : Outport
  wires:
  Switch1/1 -> Saturation/1
  Load/1 -> PI/2(Load)
  set_ISC/1 -> Switch1/2
  Switch2/1 -> Bus Selector/1
  Bus Creator1/1 -> Switch2/3
  Bus Creator2/1 -> Switch2/1
  if condition/1(Boolean) -> Switch2/2
  Constant2/1 -> Bus Creator1/1  "Load_I"
  Saturation/1 -> Load_out/1
  rotv_idle/1 -> if condition/1(rotv_idle), Subtract/1
  rotv/1 -> if condition/2(rotv), Subtract/2
  PI/1(ISCtrl.Load_I out) -> Bus Creator2/1
  Bus Selector/2 -> Switch1/1  "<Load>"
  Bus Selector/1 -> Memory1/1  "<Load_I>"
  Memory1/1 -> PI/1(ISCtrl.Load_I)
  Subtract/1 -> PI/3(drotv)  "drotv"
  PI/2(Load out) -> Bus Creator2/2
  Load Copy/1 -> Bus Creator1/2
  Load Copy2/1 -> Switch1/3

== system PTEngineCU/CarMaker/IPG Vehicle/PowerTrain/ECU Example/MyEngineCU/if Engine_on/TrqFull & TrqDrag & TrqOpt ==
  rotv : Inport
  Mappings : Inport  Port=2
  Bus Creator1 : BusCreator  Inputs=3
  Bus Selector : BusSelector  OutputSignals=TrqFull,TrqDrag,TrqOpt
  Bus Selector1 : BusSelector  OutputSignals=x,z
  Bus Selector2 : BusSelector  OutputSignals=x,z
  Bus Selector3 : BusSelector  OutputSignals=x,z
  Lookup Table Dynamic : simulink/Lookup Tables/Lookup Table Dynamic  LookUpMeth=Interpolation-Use End Values  OutDataTypeStr=float('double')  OutputDataTypeScalingMode=Specify via dialog  OutDataType=float('double')  OutScaling=2^-10  DoSatur=off
  Lookup Table Dynamic1 : simulink/Lookup Tables/Lookup Table Dynamic  LookUpMeth=Interpolation-Use End Values  OutDataTypeStr=float('double')  OutputDataTypeScalingMode=Specify via dialog  OutDataType=float('double')  OutScaling=2^-10  DoSatur=off
  Lookup Table Dynamic2 : simulink/Lookup Tables/Lookup Table Dynamic  LookUpMeth=Interpolation-Use End Values  OutDataTypeStr=float('double')  OutputDataTypeScalingMode=Specify via dialog  OutDataType=float('double')  OutScaling=2^-10  DoSatur=off
  Trg : Outport
  wires:
  Bus Selector1/1 -> Lookup Table Dynamic/2  "<x>"
  Bus Selector1/2 -> Lookup Table Dynamic/3  "<z>"
  Bus Selector/1 -> Bus Selector1/1  "<TrqFull>"
  Bus Selector/2 -> Bus Selector2/1  "<TrqDrag>"
  Bus Selector/3 -> Bus Selector3/1  "<TrqOpt>"
  Bus Selector2/2 -> Lookup Table Dynamic1/3  "<z>"
  Bus Selector2/1 -> Lookup Table Dynamic1/2  "<x>"
  Bus Selector3/1 -> Lookup Table Dynamic2/2  "<x>"
  Bus Selector3/2 -> Lookup Table Dynamic2/3  "<z>"
  Lookup Table Dynamic/1 -> Bus Creator1/1  "TrqFull"
  Lookup Table Dynamic1/1 -> Bus Creator1/2  "TrqDrag"
  Lookup Table Dynamic2/1 -> Bus Creator1/3  "TrqOpt"
  rotv/1 -> Lookup Table Dynamic/1, Lookup Table Dynamic1/1, Lookup Table Dynamic2/1
  Bus Creator1/1 -> Trg/1
  Mappings/1 -> Bus Selector/1

== system PTEngineCU/CarMaker/IPG Vehicle/PowerTrain/ECU Example/MyEngineCU/if Engine_on/FuelCutOff Function/If Action Subsystem ==
  FuelCutOff : Inport  OutDataType=sfix(16)  OutScaling=2^0
  Action Port : ActionPort  ActionType=then
  Constant : Constant  Value=0.0  OutDataType=sfix(16)  OutScaling=2^0
  FuelCutOff out : Outport  OutDataType=sfix(16)  OutScaling=2^0
  Load out : Outport  Port=2  OutDataType=sfix(16)  OutScaling=2^0  InitialOutput=0
  wires:
  Constant/1 -> Load out/1
  FuelCutOff/1 -> FuelCutOff out/1

== system PTEngineCU/CarMaker/IPG Vehicle/PowerTrain/ECU Example/MyEngineCU/if Engine_on/FuelCutOff Function/If Action Subsystem1 ==
  FuelCutOff : Inport  OutDataType=sfix(16)  OutScaling=2^0
  Load : Inport  Port=2  OutDataType=sfix(16)  OutScaling=2^0
  Action Port : ActionPort  ActionType=else
  FuelCutOff out : Outport  OutDataType=sfix(16)  OutScaling=2^0
  Load out : Outport  Port=2  OutDataType=sfix(16)  OutScaling=2^0
  wires:
  Load/1 -> Load out/1
  FuelCutOff/1 -> FuelCutOff out/1

== system PTEngineCU/CarMaker/IPG Vehicle/PowerTrain/ECU Example/MyEngineCU/if Engine_on/FuelCutOff Function/If Action Subsystem2 ==
  Load : Inport  OutDataType=sfix(16)  OutScaling=2^0
  rotv : Inport  Port=2  OutDataType=sfix(16)  OutScaling=2^0
  nFuelCutOff : Inport  Port=3  OutDataType=sfix(16)  OutScaling=2^0
  Action Port : ActionPort  ActionType=elseif
  Compare To Constant : simulink/Logic and Bit Operations/Compare To Constant  SystemSampleTime=-1  relop=<=  const=1e-3  LogicOutDataTypeMode=uint8  ZeroCross=off
  Constant : Constant  OutDataType=sfix(16)  OutScaling=2^0
  Constant1 : Constant  Value=0  OutDataType=sfix(16)  OutScaling=2^0
  Gain : Gain  ParameterDataType=sfix(16)  ParameterScaling=2^0  OutDataType=sfix(16)  OutScaling=2^0
  Logical Operator : Logic  AllPortsSameDT=off  OutDataTypeMode=boolean  OutDataTypeStr=boolean
  Relational Operator : RelationalOperator  LogicOutDataTypeMode=boolean  OutDataTypeStr=boolean
  Switch : Switch  Criteria=u2 ~= 0  OutDataType=sfix(16)  OutScaling=2^0
  FuelCutOff out : Outport  OutDataType=sfix(16)  OutScaling=2^0
  Load out : Outport  Port=2  OutDataType=sfix(16)  OutScaling=2^0
  wires:
  Load/1 -> Compare To Constant/1, Gain/1
  Switch/1 -> FuelCutOff out/1
  rotv/1 -> Relational Operator/1
  nFuelCutOff/1 -> Relational Operator/2
  Relational Operator/1 -> Logical Operator/2
  Compare To Constant/1 -> Logical Operator/1
  Logical Operator/1 -> Switch/2
  Constant/1 -> Switch/1
  Constant1/1 -> Switch/3
  Gain/1 -> Load out/1

== system PTEngineCU/CarMaker/IPG Vehicle/PowerTrain/ECU Example/MyEngineCU/if Engine_on/Idle Speed Control/PI ==
  ISCtrl.Load_I : Inport  OutDataType=sfix(16)  OutScaling=2^0
  Load : Inport  Port=2  OutDataType=sfix(16)  OutScaling=2^0
  drotv : Inport  Port=3  OutDataType=sfix(16)  OutScaling=2^0
  Add : Sum  OutDataType=sfix(16)  OutScaling=2^-10
  Add1 : Sum  OutDataType=sfix(16)  OutScaling=2^-10
  Constant : Constant  Value=0.0  OutDataType=sfix(16)  OutScaling=2^0
  If : If  IfExpression=u1 < 1e-3
  If Action Subsystem : Subsystem  TreatAsAtomicUnit=on
  If Action Subsystem1 : Subsystem  TreatAsAtomicUnit=on
  Load1 : InportShadow  Port=2  OutDataType=sfix(16)  OutScaling=2^0
  Max : MinMax  Function=max  Inputs=2  OutDataType=sfix(16)  OutScaling=2^0
  Merge : Merge
  Merge1 : Merge
  Product : Product  OutDataType=sfix(16)  OutScaling=2^0  RndMeth=Zero
  Read CM Parameter : CarMaker4SL/Read CM Parameter  xfile=Vehicle  xkey=PowerTrain.MyEngineCU.ISCtrl.P  xnout=1  xdefaults=0.1  xmuxed=on
  Saturation : Saturate  UpperLimit=1  LowerLimit=0  OutDataType=sfix(16)  OutScaling=2^0
  ISCtrl.Load_I out : Outport  OutDataType=sfix(16)  OutScaling=2^0
  Load out : Outport  Port=2  OutDataType=sfix(16)  OutScaling=2^0
  wires:
  Add/1 -> Load out/1  "Load"
  Add1/1 -> Saturation/1
  drotv/1 -> Product/1, If Action Subsystem/2(drotv), If Action Subsystem1/2(drotv)
  Read CM Parameter/1 -> Product/2
  Product/1 -> Max/1
  Max/1 -> Add1/2
  Constant/1 -> Max/2
  Load/1 -> Add/1
  ISCtrl.Load_I/1 -> If Action Subsystem/1(ISCtrl.Load_I), If Action Subsystem1/1(ISCtrl.Load_I)
  If/2 -> If Action Subsystem/Action
  Merge/1 -> Add1/1
  If Action Subsystem/2(Load_I out) -> Merge/2
  If Action Subsystem/1(ISCtrl.Load_I out) -> Merge1/2
  If/1 -> If Action Subsystem1/Action
  If Action Subsystem1/2(Load_I out) -> Merge/1
  If Action Subsystem1/1(ISCtrl.Load_I out) -> Merge1/1
  Merge1/1 -> ISCtrl.Load_I out/1  "Load_I"
  Load1/1 -> If/1
  Saturation/1 -> Add/2

== system PTEngineCU/CarMaker/IPG Vehicle/PowerTrain/ECU Example/MyEngineCU/if Engine_on/Idle Speed Control/if condition ==
  rotv_idle : Inport  OutDataType=sfix(16)  OutScaling=2^0
  rotv : Inport  Port=2
  Add : Sum  OutDataType=sfix(16)  OutScaling=2^-10
  Constant1 : Constant  Value=200.0  OutDataType=sfix(16)  OutScaling=2^0
  Relational Operator : RelationalOperator  Operator=<  LogicOutDataTypeMode=boolean  OutDataTypeStr=boolean
  rpm2radsec : Gain  Gain=0.104719755  ParameterDataType=sfix(16)  ParameterScaling=2^0  OutDataType=sfix(16)  OutScaling=2^0
  Boolean : Outport
  wires:
  rpm2radsec/1 -> Add/2
  Constant1/1 -> rpm2radsec/1
  rotv_idle/1 -> Add/1
  Relational Operator/1 -> Boolean/1
  rotv/1 -> Relational Operator/1
  Add/1 -> Relational Operator/2

== system PTEngineCU/CarMaker/IPG Vehicle/PowerTrain/ECU Example/MyEngineCU/if Engine_on/Idle Speed Control/PI/If Action Subsystem ==
  ISCtrl.Load_I : Inport  OutDataType=sfix(16)  OutScaling=2^0
  drotv : Inport  Port=2  OutDataType=sfix(16)  OutScaling=2^0
  Action Port : ActionPort  ActionType=else
  Add : Sum  OutDataType=sfix(16)  OutScaling=2^-10
  Constant : Constant  OutDataType=sfix(16)  OutScaling=2^0
  Constant1 : Constant  Value=200.0  OutDataType=sfix(16)  OutScaling=2^0
  Divide : Product  Inputs=*/  OutDataType=sfix(16)  OutScaling=2^-10
  Gain : Gain  ParameterDataType=sfix(16)  ParameterScaling=2^0  OutDataType=sfix(16)  OutScaling=2^0
  Product : Product  OutDataType=sfix(16)  OutScaling=2^0  RndMeth=Zero
  Saturation : Saturate  UpperLimit=1  LowerLimit=0  OutDataType=sfix(16)  OutScaling=2^0
  rpm2radsec : Gain  Gain=0.104719755  ParameterDataType=sfix(16)  ParameterScaling=2^0  OutDataType=sfix(16)  OutScaling=2^0
  ISCtrl.Load_I out : Outport  OutDataType=sfix(16)  OutScaling=2^0
  Load_I out : Outport  Port=2  OutDataType=sfix(16)  OutScaling=2^0
  wires:
  ISCtrl.Load_I/1 -> Product/1, Gain/1
  Product/1 -> Load_I out/1
  Add/1 -> Saturation/1  "fac"
  Constant/1 -> Add/1
  Divide/1 -> Add/2
  drotv/1 -> Divide/1
  rpm2radsec/1 -> Divide/2
  Constant1/1 -> rpm2radsec/1
  Saturation/1 -> Product/2
  Gain/1 -> ISCtrl.Load_I out/1

== system PTEngineCU/CarMaker/IPG Vehicle/PowerTrain/ECU Example/MyEngineCU/if Engine_on/Idle Speed Control/PI/If Action Subsystem1 ==
  ISCtrl.Load_I : Inport  OutDataType=sfix(16)  OutScaling=2^0
  drotv : Inport  Port=2  OutDataType=sfix(16)  OutScaling=2^0
  Action Port : ActionPort  ActionType=then
  Add : Sum  OutDataType=sfix(16)  OutScaling=2^-10
  Gain : Gain  ParameterDataType=sfix(16)  ParameterScaling=2^0  OutDataType=sfix(16)  OutScaling=2^0
  Gain1 : Gain  ParameterDataType=sfix(16)  ParameterScaling=2^0  OutDataType=sfix(16)  OutScaling=2^0
  ISCtrl_I : Constant  Value=0.01  OutDataType=fixdt(1, 16)  OutScaling=2^0
  Product : Product  OutDataType=sfix(16)  OutScaling=2^0  RndMeth=Zero
  Saturation : Saturate  UpperLimit=1  LowerLimit=0  OutDataType=sfix(16)  OutScaling=2^0
  ISCtrl.Load_I out : Outport  OutDataType=sfix(16)  OutScaling=2^0
  Load_I out : Outport  Port=2  OutDataType=sfix(16)  OutScaling=2^0
  wires:
  Add/1 -> Saturation/1
  Saturation/1 -> Gain/1, Gain1/1
  ISCtrl.Load_I/1 -> Add/2
  Product/1 -> Add/1
  drotv/1 -> Product/1
  ISCtrl_I/1 -> Product/2
  Gain/1 -> ISCtrl.Load_I out/1
  Gain1/1 -> Load_I out/1
